simulink model "Inverterf_pair_harmonics"  (R2023b)
settings: Solver=FixedStepAuto  StartTime=0.0  StopTime=Tfinal  RelTol=1e-3
InitFcn:
  | param
values from neighbouring files (symbols this model uses):
  C_DCA = 150e-6    (= 0.00015)    [param.m]
  C_DCB = 150e-6    (= 0.00015)    [param.m]
  C_DCC = 150e-6    (= 0.00015)    [param.m]
  f_motor = 1000    [param.m]
  Ld = 120e-6    (= 0.00012)    [param.m]    (also in untitled6.m = 0.5)
  Lq = 200e-6    (= 0.0002)    [param.m]    (also in untitled6.m = 1)
  LSource = 1e-6    (= 1e-06)    [param.m]
  ma = 0.9    [param.m]
  mode = 1    [param.m]
  ModuleAPhase = 0    [param.m]
  ModuleBPhase = 0    [param.m]
  ModuleCPhase = 0    [param.m]
  Rmotor = 3    [param.m]    (also in untitled6.m)
  RSource = 0.01    [param.m]
  SampleTime = 1e-8    (= 1e-08)    [param.m]
  VDC = 1070    [param.m]
undefined symbols (not defined in the file or in its folder): ESLA, ESLB, ESRA, ESRB, ESRC
libraries: spsSeriesRLCBranchLib x14, spsCurrentMeasurementLib x10, spsVoltageMeasurementLib x8, spsMosfetLib x6, simulink x6, spsTriangleGeneratorLib x3, spsVariableInductorLib x3, spsDCVoltageSourceLib x1, spspowerguiLib x1
settings Model: Creator=enesa  LastModifiedBy=enesa

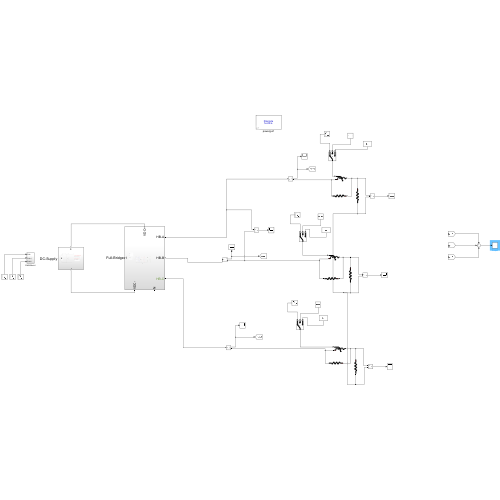
[thumbnail: Simulink's stored preview of the top-level diagram]
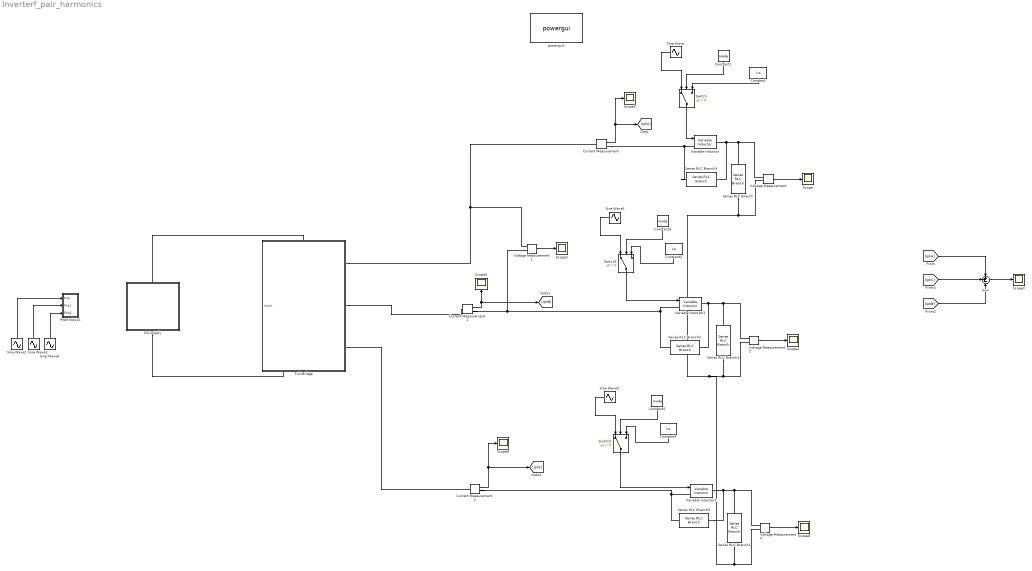
== system Inverterf_pair_harmonics ==
  Constant : Constant  Value=Lq
  Constant1 : Constant  Value=mode
  Constant2 : Constant  Value=Lq
  Constant3 : Constant  Value=mode
  Constant4 : Constant  Value=Lq
  Constant5 : Constant  Value=mode
  Current Measurement : spsCurrentMeasurementLib/Current Measurement  PhasorSimulation=off  OutputType=Complex  PSBequivalent=0
  Current Measurement1 : spsCurrentMeasurementLib/Current Measurement  PhasorSimulation=off  OutputType=Complex  PSBequivalent=0
  Current Measurement2 : spsCurrentMeasurementLib/Current Measurement  PhasorSimulation=off  OutputType=Complex  PSBequivalent=0
  DC-Supply : Subsystem
  Full-Bridge : Subsystem
      settings: PortSchema="{\"entries\":[{\"content\":{\"sides\":[{\"content\":{\"connectorIds\":[\"In1\"]},\"type\":\"ConnectorPlacement.EquallySpacedRectSide\",\"uuid\":\"92c2640b-bb56-47f8-9c41-2323b38839f8\"},{\"content\":{\"connectorIds\":[\"RConn1\",\"RConn2\",\"RConn3\"],\"side\":\"RIGHT\"},\"type\":\"ConnectorPlacement.EquallySpacedRectSide\",\"uuid\":\"0b5c90a1-e2e1-4478-84c9-834496a6568e\"},{\"content\":{\"connectorIds\":[\"LConn1\"],\"side\":\"TOP\"},\"type\":\"ConnectorPlacement.EquallySpacedRectSide\",\"uuid\":\"1c803fb0-9096-4a7d-b495-aabd35d72306\"},{\"content\":{\"connectorIds\":[\"RConn4\",\"RConn5\"],\"side\":\"BOTTOM\"},\"type\":\"ConnectorPlacement.EquallySpacedRectSide\",\"uuid\":\"5a2d766c-8c3f-4943-ab0f-0e1988e2f8d8\"},{\"content\":{\"side\":\"HIDDEN\"},\"type\":\"ConnectorPlacement.EquallySpacedRectSide\",\"uuid\":\"8868c32c-a67f-4887-a91d-dc24242eaee2\"}]},\"type\":\"ConnectorPlacement.EquallySpacedConnector\",\"uuid\":\"a3546067-6216-40b0-bae0-9d71271c5112\"}],\"packageUris\":[\"http://schema.mathworks.com/mf0/Connector/R2020b\"],\"version\":\"1.0\"}"
  PWM Block1 : Subsystem
  Scope{,1..5,8..9} (8 alike) : Scope
  Series RLC Branch : spsSeriesRLCBranchLib/Series RLC Branch  LConnTagsString=__new0  RConnTagsString=__new0  BranchType=R  Resistance=Rmotor  Inductance=1e-3  SetiL0=off  InitialCurrent=0  Capacitance=1e-6  Setx0=off  InitialVoltage=0  Measurements=None
  Series RLC Branch1 : spsSeriesRLCBranchLib/Series RLC Branch  LConnTagsString=__new0  RConnTagsString=__new0  BranchType=R  Resistance=Rmotor  Inductance=1e-3  SetiL0=off  InitialCurrent=0  Capacitance=1e-6  Setx0=off  InitialVoltage=0  Measurements=None
  Series RLC Branch2 : spsSeriesRLCBranchLib/Series RLC Branch  LConnTagsString=__new0  RConnTagsString=__new0  BranchType=R  Resistance=Rmotor  Inductance=1e-3  SetiL0=off  InitialCurrent=0  Capacitance=1e-6  Setx0=off  InitialVoltage=0  Measurements=None
  Series RLC Branch3 : spsSeriesRLCBranchLib/Series RLC Branch  LConnTagsString=__new0  RConnTagsString=__new0  BranchType=R  Resistance=10e3  Inductance=1e-3  SetiL0=off  InitialCurrent=0  Capacitance=1e-6  Setx0=off  InitialVoltage=0  Measurements=None
  Series RLC Branch4 : spsSeriesRLCBranchLib/Series RLC Branch  LConnTagsString=__new0  RConnTagsString=__new0  BranchType=R  Resistance=10e3  Inductance=1e-3  SetiL0=off  InitialCurrent=0  Capacitance=1e-6  Setx0=off  InitialVoltage=0  Measurements=None
  Series RLC Branch5 : spsSeriesRLCBranchLib/Series RLC Branch  LConnTagsString=__new0  RConnTagsString=__new0  BranchType=R  Resistance=10e3  Inductance=1e-3  SetiL0=off  InitialCurrent=0  Capacitance=1e-6  Setx0=off  InitialVoltage=0  Measurements=None
  Sine Wave : Sin  Amplitude=(Ld-Lq)/2  Bias=(Ld+Lq)/2  Frequency=2*pi*500  SampleTime=0
  Sine Wave1 : Sin  Amplitude=(Ld-Lq)/2  Bias=(Ld+Lq)/2  Frequency=2*pi*500  Phase=4*pi/3  SampleTime=0
  Sine Wave2 : Sin  Amplitude=ma  Frequency=f_motor*2*pi  SampleTime=0
  Sine Wave3 : Sin  Amplitude=ma  Frequency=f_motor*2*pi  Phase=-2*pi/3  SampleTime=0
  Sine Wave4 : Sin  Amplitude=ma  Frequency=f_motor*2*pi  Phase=2*pi/3  SampleTime=0
  Sine Wave5 : Sin  Amplitude=(Ld-Lq)/2  Bias=(Ld+Lq)/2  Frequency=2*pi*500  Phase=2*pi/3  SampleTime=0
  Sum : Sum  Inputs=++-
  Switch : Switch  Criteria=u2 > Threshold  SaturateOnIntegerOverflow=off  InputSameDT=off
  Switch1 : Switch  Criteria=u2 > Threshold  SaturateOnIntegerOverflow=off  InputSameDT=off
  Switch2 : Switch  Criteria=u2 > Threshold  SaturateOnIntegerOverflow=off  InputSameDT=off
  Variable Inductor : spsVariableInductorLib/Variable Inductor  methode=Backward Euler  Labsmin=1e-6  Initialize=off  iL0=0  L0=1e-3  Vl0=-2.9698e-14
      settings: LibrarySourceBlock=sps_lib/Passives/Variable Inductor
  Variable Inductor1 : spsVariableInductorLib/Variable Inductor  methode=Backward Euler  Labsmin=1e-6  Initialize=off  iL0=0  L0=1e-3  Vl0=2.9698e-14
      settings: LibrarySourceBlock=sps_lib/Passives/Variable Inductor
  Variable Inductor2 : spsVariableInductorLib/Variable Inductor  methode=Backward Euler  Labsmin=1e-6  Initialize=off  iL0=0  L0=1e-3  Vl0=2.2274e-14
      settings: LibrarySourceBlock=sps_lib/Passives/Variable Inductor
  Voltage Measurement{,1..2,4} (4 alike) : spsVoltageMeasurementLib/Voltage Measurement  PhasorSimulation=off  OutputType=Complex  PSBequivalent=0
  powergui1 : spspowerguiLib/powergui  Priority=1  SimulationMode=Discrete  SampleTime=SampleTime  frequency=60  Iterations=50  frequencyindice=0  Pbase=100e6  ErrMax=1e-4  UnitsV=kV  UnitsW=MW  buscounter=0  FunctionMessages=off  echomessages=off  EnableUseOfTLC=off  CurrentSourceSwitches=off  DisableSnubberDevices=off  DisableRonSwitches=off  DisableVfSwitches=off  DisplayEquations=off  AutomaticDiscreteSolvers=off  SolverType=Tustin/Backward Euler (TBE)  Interpol=off  ExternalGateDelay=off  methode=off  Ts=100  x0status=blocks  SPID=on  SwTol=0  HookPort=off  NonlinearTolerance=1e-4  nMaxIteration=100  ContinueOnMaxIteration=off  RestoreLinks=warning  ResistiveCurrentMeasurement=off  Frange=[1e3:1e3:240e3]  Ylog=off  Xlog=on  ShowGrid=off  save=off  variable=ZData  structure=ScopeData2  ZoomFFT=off  StartTime=0.02  cycles=400  DisplayStyle=2  fundamental=80e3  FreqAxis=off  MaxFrequency=240e3  frequencyindicesteady=1  RmsSteady=1  display=off
  wires:
  Current Measurement/1 -> [IphA], Scope1/1
  Sine Wave/1 -> Switch/1
  Voltage Measurement/1 -> Scope/1
  Current Measurement1/1 -> Scope5/1, [IphB]
  Voltage Measurement2/1 -> Scope4/1
  Current Measurement2/1 -> [IphC], Scope9/1
  Voltage Measurement4/1 -> Scope8/1
  Constant/1 -> Switch/3
  Switch/1 -> Variable Inductor/1
  Constant1/1 -> Switch/2
  Sine Wave2/1 -> PWM Block1/1(PhA)
  Sine Wave4/1 -> PWM Block1/3(PhA2)
  Sine Wave3/1 -> PWM Block1/2(PhA1)
  Constant3/1 -> Switch1/2
  Constant2/1 -> Switch1/3
  Switch1/1 -> Variable Inductor1/1
  Sine Wave1/1 -> Switch1/1
  Constant5/1 -> Switch2/2
  Sine Wave5/1 -> Switch2/1
  Switch2/1 -> Variable Inductor2/1
  Constant4/1 -> Switch2/3
  Voltage Measurement1/1 -> Scope2/1
  [IphA] -> Sum/1
  [IphB] -> Sum/3
  [IphC] -> Sum/2
  Sum/1 -> Scope3/1
  connections:
  Variable Inductor/RConn1 -- Series RLC Branch3/LConn1 -- Series RLC Branch/LConn1 -- Voltage Measurement/LConn1
  Current Measurement/RConn1 -- Series RLC Branch3/RConn1 -- Variable Inductor/LConn1
  Voltage Measurement2/LConn1 -- Series RLC Branch4/LConn1 -- Variable Inductor1/RConn1 -- Series RLC Branch1/LConn1
  Current Measurement1/RConn1 -- Variable Inductor1/LConn1 -- Series RLC Branch4/RConn1 -- Voltage Measurement1/LConn2
  Series RLC Branch/RConn1 -- Series RLC Branch2/RConn1 -- Voltage Measurement4/LConn2 -- Voltage Measurement2/LConn2 -- Series RLC Branch1/RConn1 -- Voltage Measurement/LConn2
  Voltage Measurement4/LConn1 -- Series RLC Branch5/LConn1 -- Variable Inductor2/RConn1 -- Series RLC Branch2/LConn1
  Current Measurement2/RConn1 -- Series RLC Branch5/RConn1 -- Variable Inductor2/LConn1
  DC-Supply/RConn1 -- Full-Bridge/RConn4
  DC-Supply/LConn1 -- Full-Bridge/LConn1
  Full-Bridge/RConn3 -- Current Measurement2/LConn1
  Full-Bridge/RConn1 -- Voltage Measurement1/LConn1 -- Current Measurement/LConn1
  Full-Bridge/RConn2 -- Current Measurement1/LConn1

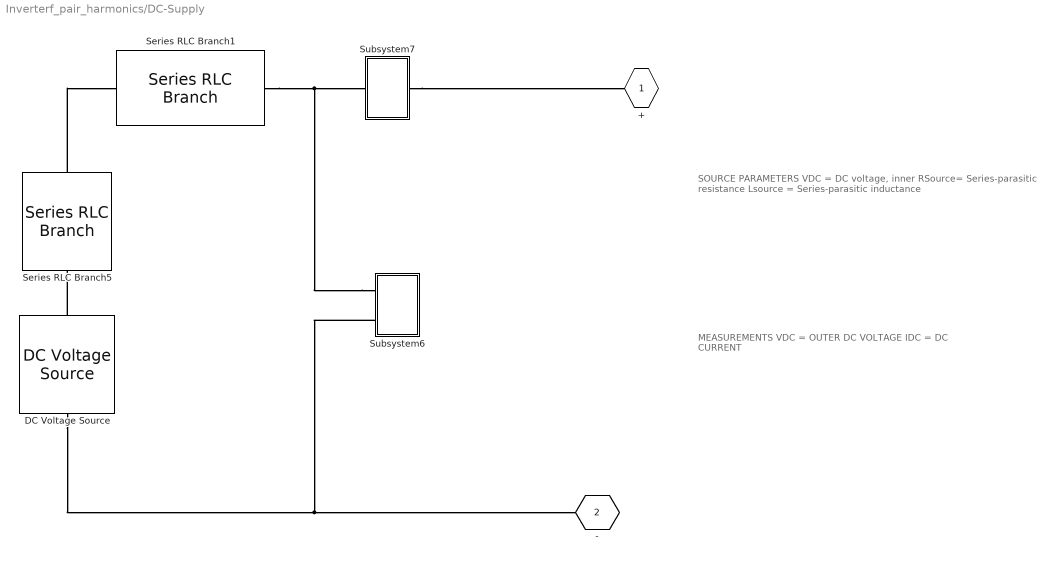
== system Inverterf_pair_harmonics/DC-Supply ==
  note: SOURCE PARAMETERS
      | VDC = DC voltage, inner
      | RSource= Series-parasitic resistance
      | Lsource = Series-parasitic inductance
  note: MEASUREMENTS
      | VDC = OUTER DC VOLTAGE
      | IDC = DC CURRENT
  DC Voltage Source : spsDCVoltageSourceLib/DC Voltage Source  Amplitude=VDC  Measurements=None
  Series RLC Branch1 : spsSeriesRLCBranchLib/Series RLC Branch  LConnTagsString=__new0  RConnTagsString=__new0  BranchType=L  Resistance=LSource  Inductance=LSource  SetiL0=off  InitialCurrent=0  Capacitance=0.01  Setx0=off  InitialVoltage=0  Measurements=None
  Series RLC Branch5 : spsSeriesRLCBranchLib/Series RLC Branch  LConnTagsString=__new0  RConnTagsString=__new0  BranchType=R  Resistance=RSource  Inductance=ESLA  SetiL0=off  InitialCurrent=0  Capacitance=0.01  Setx0=off  InitialVoltage=0  Measurements=None
  Subsystem6 : Subsystem
  Subsystem7 : Subsystem
  + : PMIOPort  Side=Left
  - : PMIOPort  Port=2  Side=Right
  connections:
  Series RLC Branch5/LConn1 -- Series RLC Branch1/RConn1
  DC Voltage Source/LConn1 -- Subsystem6/LConn2 -- -/RConn1
  Subsystem6/LConn1 -- Series RLC Branch1/LConn1 -- Subsystem7/RConn1
  DC Voltage Source/RConn1 -- Series RLC Branch5/RConn1
  Subsystem7/LConn1 -- +/RConn1

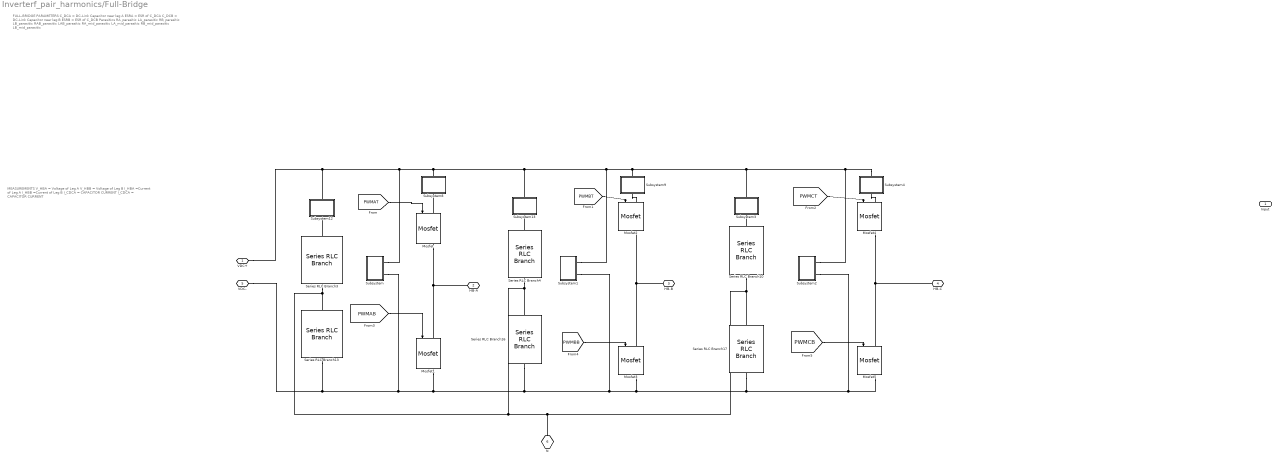
== system Inverterf_pair_harmonics/Full-Bridge ==
  note: MEASUREMENTS
      | V_HBA = Voltage of Leg A
      | V_HBB = Voltage of Leg B
      | I_HBA =Current of Leg A
      | I_HBB =Current of Leg B
      | I_CDCA = CAPACITOR CURRENT
      | I_CDCA = CAPACITOR CURRENT
  note: FULL-BRIDGE PARAMETERS
      | C_DCA = DC-Link Capacitor near leg A
      | ESRA = ESR of C_DCA
      | C_DCB = DC-Link Capacitor near leg B
      | ESRB = ESR of C_DCB
      | Parasitics
      | RA_parasitic
      | LA_parasitic
      | RB_parasitic
      | LB_parasitic
      | RAB_parasitic
      | LAB_parasitic
      | RA_mid_parasitic
      | LA_mid_parasitic
      | RB_mid_parasitic
      | LB_mid_parasitic
  Input : Inport
  Mosfet{,1..5} (6 alike) : spsMosfetLib/Mosfet  Ron=0.1  Lon=0  Rd=0.01  Vfd=0  IC=0  Rs=1e5  Cs=inf  Measurements=on
  Series RLC Branch10 : spsSeriesRLCBranchLib/Series RLC Branch  LConnTagsString=__new0  RConnTagsString=__new0  BranchType=C  Resistance=ESRC  Inductance=ESLB  SetiL0=off  InitialCurrent=0  Capacitance=C_DCC  Setx0=off  InitialVoltage=0  Measurements=None
  Series RLC Branch13 : spsSeriesRLCBranchLib/Series RLC Branch  LConnTagsString=__new0  RConnTagsString=__new0  BranchType=C  Resistance=ESRA  Inductance=ESLA  SetiL0=off  InitialCurrent=0  Capacitance=C_DCA  Setx0=off  InitialVoltage=0  Measurements=None
  Series RLC Branch16 : spsSeriesRLCBranchLib/Series RLC Branch  LConnTagsString=__new0  RConnTagsString=__new0  BranchType=C  Resistance=ESRB  Inductance=ESLB  SetiL0=off  InitialCurrent=0  Capacitance=C_DCB  Setx0=off  InitialVoltage=0  Measurements=None
  Series RLC Branch17 : spsSeriesRLCBranchLib/Series RLC Branch  LConnTagsString=__new0  RConnTagsString=__new0  BranchType=C  Resistance=ESRB  Inductance=ESLB  SetiL0=off  InitialCurrent=0  Capacitance=C_DCB  Setx0=off  InitialVoltage=0  Measurements=None
  Series RLC Branch3 : spsSeriesRLCBranchLib/Series RLC Branch  LConnTagsString=__new0  RConnTagsString=__new0  BranchType=C  Resistance=ESRA  Inductance=ESLA  SetiL0=off  InitialCurrent=0  Capacitance=C_DCA  Setx0=off  InitialVoltage=0  Measurements=None
  Series RLC Branch4 : spsSeriesRLCBranchLib/Series RLC Branch  LConnTagsString=__new0  RConnTagsString=__new0  BranchType=C  Resistance=ESRB  Inductance=ESLB  SetiL0=off  InitialCurrent=0  Capacitance=C_DCB  Setx0=off  InitialVoltage=0  Measurements=None
  Subsystem : Subsystem
  Subsystem1 : Subsystem
  Subsystem12 : Subsystem
  Subsystem13 : Subsystem
  Subsystem2 : Subsystem
  Subsystem3 : Subsystem
  Subsystem4 : Subsystem
  Subsystem8 : Subsystem
  Subsystem9 : Subsystem
  VDC+ : PMIOPort  Side=Left
  HB-A : PMIOPort  Port=2  Side=Right
  HB-B : PMIOPort  Port=3  Side=Right
  HB-C : PMIOPort  Port=4  Side=Right
  VDC- : PMIOPort  Port=5  Side=Right
  N : PMIOPort  Port=6  Side=Right
  wires:
  [PWMAB] -> Mosfet1/1
  [PWMAT] -> Mosfet/1
  [PWMBB] -> Mosfet3/1
  [PWMBT] -> Mosfet2/1
  [PWMCT] -> Mosfet4/1
  [PWMCB] -> Mosfet5/1
  connections:
  HB-A/RConn1 -- Mosfet1/LConn1 -- Mosfet/RConn1
  Subsystem9/LConn1 -- Mosfet2/LConn1
  Series RLC Branch4/LConn1 -- Subsystem13/LConn1
  Series RLC Branch3/LConn1 -- Subsystem12/LConn1
  Mosfet/LConn1 -- Subsystem8/LConn1
  Subsystem4/RConn1 -- Subsystem13/RConn1 -- VDC+/RConn1 -- Subsystem12/RConn1 -- Subsystem/LConn1 -- Subsystem8/RConn1 -- Subsystem1/LConn1 -- Subsystem9/RConn1 -- Subsystem3/RConn1 -- Subsystem2/LConn1
  Series RLC Branch10/LConn1 -- Subsystem3/LConn1
  HB-C/RConn1 -- Mosfet5/LConn1 -- Mosfet4/RConn1
  Subsystem4/LConn1 -- Mosfet4/LConn1
  Series RLC Branch10/RConn1 -- Series RLC Branch16/LConn1 -- Series RLC Branch4/RConn1 -- Series RLC Branch13/LConn1 -- Series RLC Branch3/RConn1 -- N/RConn1 -- Series RLC Branch17/LConn1
  Series RLC Branch13/RConn1 -- Series RLC Branch16/RConn1 -- Series RLC Branch17/RConn1 -- Subsystem2/LConn2 -- Mosfet5/RConn1 -- Mosfet3/RConn1 -- Subsystem1/LConn2 -- Mosfet1/RConn1 -- Subsystem/LConn2 -- VDC-/RConn1
  HB-B/RConn1 -- Mosfet3/LConn1 -- Mosfet2/RConn1

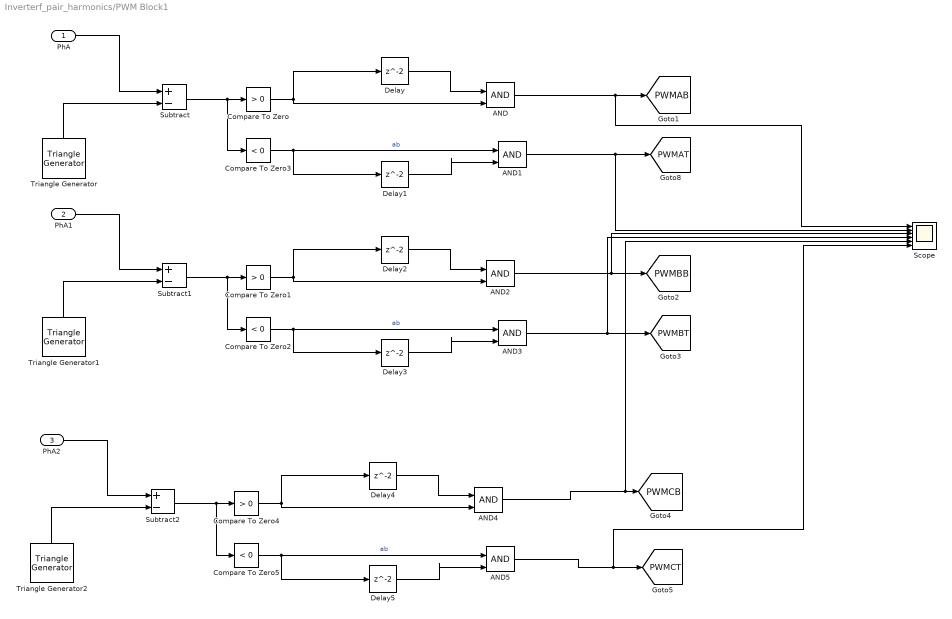
== system Inverterf_pair_harmonics/PWM Block1 ==
  PhA : Inport
  PhA1 : Inport  Port=2
  PhA2 : Inport  Port=3
  AND{,1..5} (6 alike) : Logic  IconShape=distinctive  AllPortsSameDT=off  OutDataTypeStr=boolean
  Compare To Zero : simulink/Logic and Bit Operations/Compare To Zero  relop=>  OutDataTypeStr=boolean
  Compare To Zero1 : simulink/Logic and Bit Operations/Compare To Zero  relop=>  OutDataTypeStr=boolean
  Compare To Zero2 : simulink/Logic and Bit Operations/Compare To Zero  relop=<  OutDataTypeStr=boolean
  Compare To Zero3 : simulink/Logic and Bit Operations/Compare To Zero  relop=<  OutDataTypeStr=boolean
  Compare To Zero4 : simulink/Logic and Bit Operations/Compare To Zero  relop=>  OutDataTypeStr=boolean
  Compare To Zero5 : simulink/Logic and Bit Operations/Compare To Zero  relop=<  OutDataTypeStr=boolean
  Delay{,1..5} (6 alike) : Delay
  Scope : Scope  NumInputPorts=6
  Subtract : Sum  Inputs=+-
  Subtract1 : Sum  Inputs=+-
  Subtract2 : Sum  Inputs=+-
  Triangle Generator : spsTriangleGeneratorLib/Triangle Generator  Freq=fsw  Phase=ModuleAPhase  Ts=SampleTime
  Triangle Generator1 : spsTriangleGeneratorLib/Triangle Generator  Freq=fsw  Phase=ModuleBPhase  Ts=SampleTime
  Triangle Generator2 : spsTriangleGeneratorLib/Triangle Generator  Freq=fsw  Phase=ModuleCPhase  Ts=SampleTime
  tag scope: PWMAB=global, PWMAT=global, PWMBB=global, PWMBT=global, PWMCB=global, PWMCT=global
  wires:
  PhA/1 -> Subtract/1
  Triangle Generator/1 -> Subtract/2
  Subtract/1 -> Compare To Zero3/1, Compare To Zero/1
  Compare To Zero/1 -> Delay/1, AND/2
  Delay/1 -> AND/1
  Compare To Zero3/1 -> Delay1/1, AND1/1  "ab"
  Delay1/1 -> AND1/2
  AND2/1 -> Scope/3, [PWMBB]
  AND/1 -> Scope/1, [PWMAB]
  AND4/1 -> Scope/5, [PWMCB]
  Delay3/1 -> AND3/2
  Compare To Zero1/1 -> Delay2/1, AND2/2
  Delay2/1 -> AND2/1
  Compare To Zero2/1 -> Delay3/1, AND3/1  "ab"
  Subtract1/1 -> Compare To Zero2/1, Compare To Zero1/1
  Triangle Generator1/1 -> Subtract1/2
  PhA1/1 -> Subtract1/1
  Delay5/1 -> AND5/2
  Compare To Zero4/1 -> Delay4/1, AND4/2
  Delay4/1 -> AND4/1
  Compare To Zero5/1 -> Delay5/1, AND5/1  "ab"
  Subtract2/1 -> Compare To Zero5/1, Compare To Zero4/1
  Triangle Generator2/1 -> Subtract2/2
  PhA2/1 -> Subtract2/1
  AND1/1 -> Scope/2, [PWMAT]
  AND3/1 -> Scope/4, [PWMBT]
  AND5/1 -> Scope/6, [PWMCT]

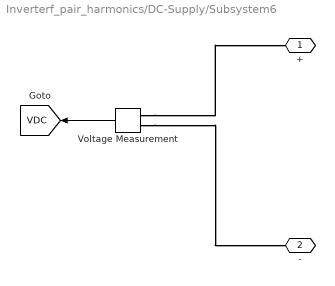
== system Inverterf_pair_harmonics/DC-Supply/Subsystem6 ==
  Voltage Measurement : spsVoltageMeasurementLib/Voltage Measurement  PhasorSimulation=off  OutputType=Complex  PSBequivalent=0
  + : PMIOPort  Side=Left
  - : PMIOPort  Port=2  Side=Left
  tag scope: VDC=global
  wires:
  Voltage Measurement/1 -> [VDC]
  connections:
  Voltage Measurement/LConn1 -- +/RConn1
  Voltage Measurement/LConn2 -- -/RConn1

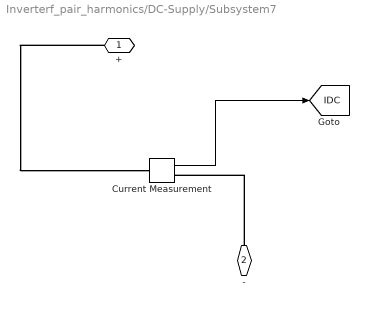
== system Inverterf_pair_harmonics/DC-Supply/Subsystem7 ==
  Current Measurement : spsCurrentMeasurementLib/Current Measurement  PhasorSimulation=off  OutputType=Complex  PSBequivalent=0
  + : PMIOPort  Side=Right
  - : PMIOPort  Port=2  Side=Left
  tag scope: IDC=global
  wires:
  Current Measurement/1 -> [IDC]
  connections:
  +/RConn1 -- Current Measurement/LConn1
  -/RConn1 -- Current Measurement/RConn1

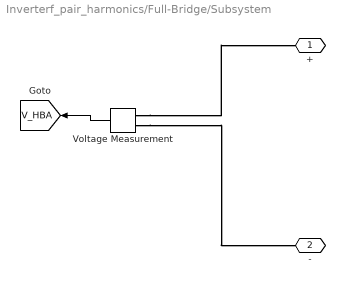
== system Inverterf_pair_harmonics/Full-Bridge/Subsystem ==
  Voltage Measurement : spsVoltageMeasurementLib/Voltage Measurement  PhasorSimulation=off  OutputType=Complex  PSBequivalent=0
  + : PMIOPort  Side=Left
  - : PMIOPort  Port=2  Side=Left
  tag scope: V_HBA=global
  wires:
  Voltage Measurement/1 -> [V_HBA]
  connections:
  Voltage Measurement/LConn1 -- +/RConn1
  Voltage Measurement/LConn2 -- -/RConn1

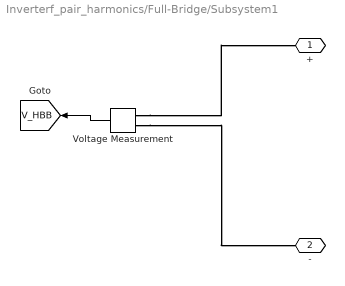
== system Inverterf_pair_harmonics/Full-Bridge/Subsystem1 ==
  Voltage Measurement : spsVoltageMeasurementLib/Voltage Measurement  PhasorSimulation=off  OutputType=Complex  PSBequivalent=0
  + : PMIOPort  Side=Left
  - : PMIOPort  Port=2  Side=Left
  tag scope: V_HBB=global
  wires:
  Voltage Measurement/1 -> [V_HBB]
  connections:
  Voltage Measurement/LConn1 -- +/RConn1
  Voltage Measurement/LConn2 -- -/RConn1

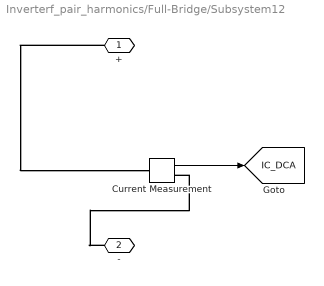
== system Inverterf_pair_harmonics/Full-Bridge/Subsystem12 ==
  Current Measurement : spsCurrentMeasurementLib/Current Measurement  PhasorSimulation=off  OutputType=Complex  PSBequivalent=0
  + : PMIOPort  Side=Right
  - : PMIOPort  Port=2  Side=Left
  tag scope: IC_DCA=global
  wires:
  Current Measurement/1 -> [IC_DCA]
  connections:
  +/RConn1 -- Current Measurement/LConn1
  -/RConn1 -- Current Measurement/RConn1

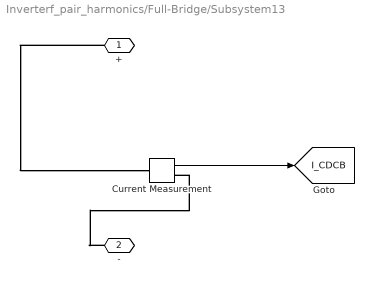
== system Inverterf_pair_harmonics/Full-Bridge/Subsystem13 ==
  Current Measurement : spsCurrentMeasurementLib/Current Measurement  PhasorSimulation=off  OutputType=Complex  PSBequivalent=0
  + : PMIOPort  Side=Right
  - : PMIOPort  Port=2  Side=Left
  tag scope: I_CDCB=global
  wires:
  Current Measurement/1 -> [I_CDCB]
  connections:
  +/RConn1 -- Current Measurement/LConn1
  -/RConn1 -- Current Measurement/RConn1

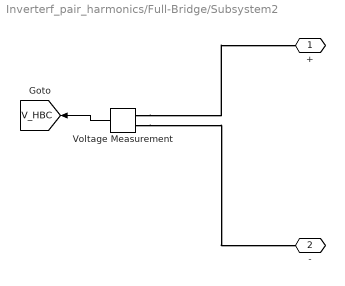
== system Inverterf_pair_harmonics/Full-Bridge/Subsystem2 ==
  Voltage Measurement : spsVoltageMeasurementLib/Voltage Measurement  PhasorSimulation=off  OutputType=Complex  PSBequivalent=0
  + : PMIOPort  Side=Left
  - : PMIOPort  Port=2  Side=Left
  tag scope: V_HBC=global
  wires:
  Voltage Measurement/1 -> [V_HBC]
  connections:
  Voltage Measurement/LConn1 -- +/RConn1
  Voltage Measurement/LConn2 -- -/RConn1

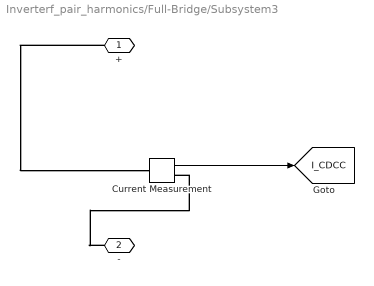
== system Inverterf_pair_harmonics/Full-Bridge/Subsystem3 ==
  Current Measurement : spsCurrentMeasurementLib/Current Measurement  PhasorSimulation=off  OutputType=Complex  PSBequivalent=0
  + : PMIOPort  Side=Right
  - : PMIOPort  Port=2  Side=Left
  tag scope: I_CDCC=global
  wires:
  Current Measurement/1 -> [I_CDCC]
  connections:
  +/RConn1 -- Current Measurement/LConn1
  -/RConn1 -- Current Measurement/RConn1

== system Inverterf_pair_harmonics/Full-Bridge/Subsystem4 ==
  Current Measurement : spsCurrentMeasurementLib/Current Measurement  PhasorSimulation=off  OutputType=Complex  PSBequivalent=0
  + : PMIOPort  Side=Right
  - : PMIOPort  Port=2  Side=Left
  tag scope: I_HBC=global
  wires:
  Current Measurement/1 -> [I_HBC]
  connections:
  +/RConn1 -- Current Measurement/LConn1
  -/RConn1 -- Current Measurement/RConn1

== system Inverterf_pair_harmonics/Full-Bridge/Subsystem8 ==
  Current Measurement : spsCurrentMeasurementLib/Current Measurement  PhasorSimulation=off  OutputType=Complex  PSBequivalent=0
  + : PMIOPort  Side=Right
  - : PMIOPort  Port=2  Side=Left
  tag scope: I_HBA=global
  wires:
  Current Measurement/1 -> [I_HBA]
  connections:
  +/RConn1 -- Current Measurement/LConn1
  -/RConn1 -- Current Measurement/RConn1

== system Inverterf_pair_harmonics/Full-Bridge/Subsystem9 ==
  Current Measurement : spsCurrentMeasurementLib/Current Measurement  PhasorSimulation=off  OutputType=Complex  PSBequivalent=0
  + : PMIOPort  Side=Right
  - : PMIOPort  Port=2  Side=Left
  tag scope: I_HBB=global
  wires:
  Current Measurement/1 -> [I_HBB]
  connections:
  +/RConn1 -- Current Measurement/LConn1
  -/RConn1 -- Current Measurement/RConn1
